simulink model "Task_3"  (R2015a)
settings: Solver=ode45  StartTime=0.0  StopTime=10.0  RelTol=1e-3
settings Model: Creator=acer  LastModifiedBy=acer

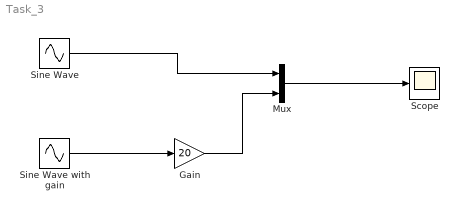
== system Task_3 ==
  Gain : Gain  Gain=20
  Mux : Mux  Inputs=2
  Scope : Scope
      settings: ShowLegends=on
  Sine Wave : Sin  SampleTime=0
  "Sine Wave with gain " : Sin  SampleTime=0
  wires:
  "Sine Wave with gain "/1 -> Gain/1
  Gain/1 -> Mux/2
  Sine Wave/1 -> Mux/1
  Mux/1 -> Scope/1
